simulink model "DragModelSquared"  (R2018b)
settings: Solver=VariableStepAuto  StartTime=0.0  StopTime=10.0  RelTol=1e-3  EnableMultiTasking=on
settings Model: Creator=jban039  LastModifiedBy=jban039
settings DataIOCC: LimitDataPoints=on
settings OptimizationCC: LifeSpan=inf
settings DebuggingCC: AllowSymbolicDim=off  SFUnexpectedBacktrackingDiag=warning  SFNoUnconditionalDefaultTransitionDiag=warning  SFExecutionAtInitializationDiag=none
settings ModelReferenceCC: PropagateSignalLabelsOutOfModel=off
settings SFSimCC: SimUseLocalCustomCode=off
settings RTWCC: RTWUseLocalCustomCode=off
settings CodeAppCC: StateflowObjectComments=on
settings GRTTargetCC: TargetLangStandard=C89/C90 (ANSI)
settings ConfigComp: CovMetricSettings=dw  CovHtmlReporting=on  CovSaveCumulativeToWorkspaceVar=on  CovSaveSingleToWorkspaceVar=on  CovExternalEMLEnable=off

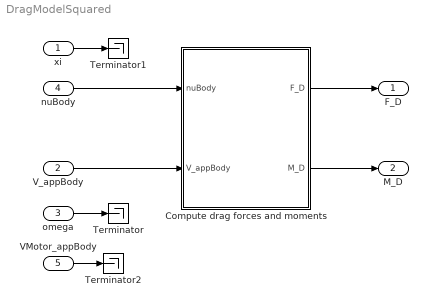
== system DragModelSquared ==
  xi : Inport  PortDimensions=3
  V_appBody : Inport  Port=2  PortDimensions=3
  omega : Inport  Port=3  PortDimensions=Uav.N_ROTORS
  nuBody : Inport  Port=4  PortDimensions=3
  VMotor_appBody : Inport  Port=5  PortDimensions=[3,4]
  Compute drag forces and moments : MATLAB Function  TreatAsAtomicUnit=on
  Terminator : Terminator
  Terminator1 : Terminator
  Terminator2 : Terminator
  F_D : Outport
  M_D : Outport  Port=2
  wires:
  Compute drag forces and moments/1(F_D) -> F_D/1
  Compute drag forces and moments/2(M_D) -> M_D/1
  V_appBody/1 -> Compute drag forces and moments/2(V_appBody)
  omega/1 -> Terminator/1
  xi/1 -> Terminator1/1
  nuBody/1 -> Compute drag forces and moments/1(nuBody)
  VMotor_appBody/1 -> Terminator2/1

== matlab function DragModelSquared/Compute drag forces and moments ==
  data: nuBody input; V_appBody input; F_D output; M_D output; Uav parameter
function [F_D, M_D] = computeDrag(nuBody, V_appBody, Uav)
%#codegen

% Calculate drag force
F_D = 0.5 * Uav.RHO_AIR * Uav.C_D * (norm(V_appBody) .* V_appBody);

% Drag moment, applied to independent axes
M_D = 0.5 * Uav.RHO_AIR * Uav.C_DM * (norm(nuBody) .* nuBody);
